simulink model "VSC_GFo_Variable_Frequency_LCL"  (R2017b)
settings: Solver=ode1  StartTime=0.0  StopTime=8  FixedStep=Time_Step  MaxStep=1e-5  RelTol=1e-3
PreLoadFcn:
  | VSC_GFo_Init;
InitFcn:
  | VSC_GFo_Init;
values from neighbouring files (symbols this model uses):
  DX_DR = 5    [VSC_GFo_Init.m]
  fb = fn    (= 50)    [VSC_GFo_Init.m]    (also in VSC_GFo_Init_v1.m; VSC_GFo_Init_wi_LCL.m)
  fn = 50    [VSC_GFo_Init.m]    (also in VSC_GFo_Init_v1.m; VSC_GFo_Init_wi_LCL.m)
  GRD00_H = 5    [VSC_GFo_Init.m]    (also in VSC_GFo_Init_v1.m; VSC_GFo_Init_wi_LCL.m)
  GRD00_Lg = GRD00_Xg/wb    (= 0.0254647908947)    [VSC_GFo_Init.m]    (also in VSC_GFo_Init_v1.m; VSC_GFo_Init_wi_LCL.m)
  GRD00_R = 4/100    (= 0.04)    [VSC_GFo_Init.m]    (also in VSC_GFo_Init_v1.m; VSC_GFo_Init_wi_LCL.m)
  GRD00_Rg = GRD00_Rg_pu*GRD00_Zb    (= 0.8)    [VSC_GFo_Init.m]    (also in VSC_GFo_Init_v1.m; VSC_GFo_Init_wi_LCL.m)
  GRD00_TD = 6    [VSC_GFo_Init.m]    (also in VSC_GFo_Init_v1.m = 2; VSC_GFo_Init_wi_LCL.m = 2)
  GRD00_TN = 1    [VSC_GFo_Init.m]    (also in VSC_GFo_Init_v1.m; VSC_GFo_Init_wi_LCL.m)
  GRD00_Ub = GRD00_Un    (= 400000)    [VSC_GFo_Init.m]    (also in VSC_GFo_Init_v1.m; VSC_GFo_Init_wi_LCL.m)
  I_thresh_pu = 1    [VSC_GFo_Init.m]
  Kp_Rvi_pu = 0.676    [VSC_GFo_Init.m]
  Time_Step = 40e-6    (= 4e-05)    [VSC_GFo_Init.m]    (also in VSC_GFo_Init_v1.m; VSC_GFo_Init_wi_LCL.m)
  VSC01_Cf = VSC01_Cf_pu * VSC01_Cb    [VSC_GFo_Init.m]    (also in VSC_GFo_Init_wi_LCL.m)
  VSC01_Cf_pu = 0.066    [VSC_GFo_Init.m]    (also in VSC_GFo_Init_wi_LCL.m)
  VSC01_Delta_P_Time_Step = 0.2    [VSC_GFo_Init.m]    (also in VSC_GFo_Init_v1.m; VSC_GFo_Init_wi_LCL.m)
  VSC01_Delta_P_Value = 0    [VSC_GFo_Init.m]    (also in VSC_GFo_Init_v1.m = 0.2; VSC_GFo_Init_wi_LCL.m = 0.2)
  VSC01_Lf = VSC01_Lf_pu * VSC01_Lb    [VSC_GFo_Init.m]    (also in VSC_GFo_Init_wi_LCL.m)
  VSC01_Lf_pu = 0.15    [VSC_GFo_Init.m]    (also in VSC_GFo_Init_wi_LCL.m)
  VSC01_Lt_pu = 0.15    [VSC_GFo_Init.m]    (also in VSC_GFo_Init_v1.m; VSC_GFo_Init_wi_LCL.m)
  VSC01_mp1 = 0.0043    [VSC_GFo_Init.m]    (also in VSC_GFo_Init_v1.m; VSC_GFo_Init_wi_LCL.m)
  VSC01_mp2 = 0.003    [VSC_GFo_Init.m]    (also in VSC_GFo_Init_v1.m = 0.0033; VSC_GFo_Init_wi_LCL.m = 0.0033)
  VSC01_mp3 = 0.04    [VSC_GFo_Init.m]    (also in VSC_GFo_Init_v1.m; VSC_GFo_Init_wi_LCL.m)
  VSC01_Pn = 1000 * 1e6    (= 1000000000)    [VSC_GFo_Init.m]    (also in VSC_GFo_Init_v1.m; VSC_GFo_Init_wi_LCL.m)
  VSC01_R = 4/100    (= 0.04)    [VSC_GFo_Init.m]    (also in VSC_GFo_Init_v1.m; VSC_GFo_Init_wi_LCL.m)
  VSC01_Rf = VSC01_Rf_pu * VSC01_Zb    [VSC_GFo_Init.m]    (also in VSC_GFo_Init_wi_LCL.m)
  VSC01_Rf_pu = 0.005    [VSC_GFo_Init.m]    (also in VSC_GFo_Init_wi_LCL.m)
  VSC01_Rt_pu = 0.005    [VSC_GFo_Init.m]    (also in VSC_GFo_Init_v1.m; VSC_GFo_Init_wi_LCL.m)
  VSC01_Rv = 0.09    [VSC_GFo_Init.m]    (also in VSC_GFo_Init_v1.m; VSC_GFo_Init_wi_LCL.m)
  VSC01_Sn = VSC01_Pn/VSC01_cosPhi_n    [VSC_GFo_Init.m]    (also in VSC_GFo_Init_v1.m; VSC_GFo_Init_wi_LCL.m)
  VSC01_T1 = 0.121    [VSC_GFo_Init.m]    (also in VSC_GFo_Init_v1.m; VSC_GFo_Init_wi_LCL.m)
  VSC01_T2 = 0.022    [VSC_GFo_Init.m]    (also in VSC_GFo_Init_v1.m; VSC_GFo_Init_wi_LCL.m)
  VSC01_Tr_PLL = 0.010    (= 0.01)    [VSC_GFo_Init.m]    (also in VSC_GFo_Init_v1.m; VSC_GFo_Init_wi_LCL.m)
  VSC01_Udc_n = 640 * 1e3    (= 640000)    [VSC_GFo_Init.m]    (also in VSC_GFo_Init_v1.m; VSC_GFo_Init_wi_LCL.m)
  VSC01_Udcb = VSC01_Udc_n    (= 640000)    [VSC_GFo_Init.m]    (also in VSC_GFo_Init_v1.m; VSC_GFo_Init_wi_LCL.m)
  VSC01_Un1 = 320 * 1e3    (= 320000)    [VSC_GFo_Init.m]    (also in VSC_GFo_Init_v1.m; VSC_GFo_Init_wi_LCL.m)
  VSC01_Un2 = 400 * 1e3    (= 400000)    [VSC_GFo_Init.m]    (also in VSC_GFo_Init_v1.m; VSC_GFo_Init_wi_LCL.m)
  VSC01_W_LF = 60    [VSC_GFo_Init.m]    (also in VSC_GFo_Init_v1.m; VSC_GFo_Init_wi_LCL.m)
  VSC01_wc1 = wb/10    (= 31.4159265359)    [VSC_GFo_Init.m]    (also in VSC_GFo_Init_v1.m; VSC_GFo_Init_wi_LCL.m)
  VSC01_wc2 = 33.3    [VSC_GFo_Init.m]    (also in VSC_GFo_Init_v1.m; VSC_GFo_Init_wi_LCL.m)
  VSC01_wc3 = 2.5    [VSC_GFo_Init.m]    (also in VSC_GFo_Init_v1.m; VSC_GFo_Init_wi_LCL.m)
undefined symbols (not defined in the file or in its folder): C_line, VSC01_id0
libraries: powerlib x29, simulink x1, powerlib_meascontrol x1
(part 1 of 2)
settings Model: Creator=Frederic_Colas  LastModifiedBy=Frederic_Colas
settings OptimizationCC: LifeSpan=inf
settings DebuggingCC: UnconnectedInputMsg=none  UnconnectedOutputMsg=none  UnconnectedLineMsg=none  SFExecutionAtInitializationDiag=none
settings HardwareCC: ProdBitPerSizeT=32  ProdBitPerPtrDiffT=32  ProdWordSize=32  ProdHWDeviceType=Specified
settings CodeAppCC: StateflowObjectComments=on
settings SimscapeCC: SimscapeNormalizeSystem=off

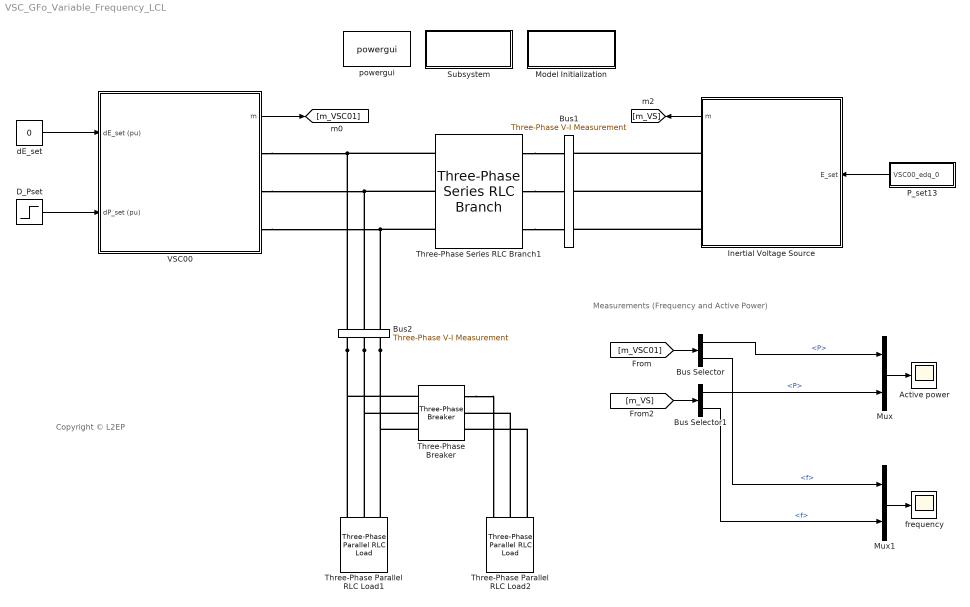
== system VSC_GFo_Variable_Frequency_LCL ==
  note: Measurements (Frequency and Active Power)
  note: Copyright © L2EP
  Active power : Scope
  Bus Selector : BusSelector  OutputSignals=control.P,control.f
  Bus Selector1 : BusSelector  OutputSignals=P,f
  Bus1 : powerlib/Measurements/Three-Phase V-I Measurement  VoltageMeasurement=no  SetLabelV=off  LabelV=Vabc  Vpu=off  VpuLL=off  CurrentMeasurement=no  SetLabelI=off  LabelI=Iabc  Ipu=off  Pbase=1e9  Vbase=VSC01_Un2  OutputType=Complex  PhasorSimulation=off  PSBequivalent=0
  "Bus2 " : powerlib/Measurements/Three-Phase V-I Measurement  VoltageMeasurement=no  SetLabelV=off  LabelV=Vabc  Vpu=off  VpuLL=off  CurrentMeasurement=no  SetLabelI=off  LabelI=Iabc  Ipu=off  Pbase=100e6  Vbase=500e3  OutputType=Complex  PhasorSimulation=off  PSBequivalent=0
  D_Pset : Step  Time=VSC01_Delta_P_Time_Step  After=VSC01_Delta_P_Value  SampleTime=0
  Inertial Voltage Source : Subsystem  mask(Inertial_Voltage_source){fb=fb, Sc=1e9, Ub=GRD00_Ub, H_eq=GRD00_H, Droop=GRD00_R, TN=GRD00_TN, TD=GRD00_TD, P0=-0.39869}
      mask prompts: fb "Nominal Frequency (Hz)"; Sc "Nominal Power (VA)"; Ub "Nominal Voltage (V)"; H_eq "Inertial Constant H (s)"; Droop "Droop Gain"; TN "Lead Time Constant"; TD "Lag Time Constant"; P0 "Initial Power"
      mask init:
      | % Update Name of LF bus for internal purpose
      |     NameStr = [get_param(gcb,'Name')];% '_LF'];
      |     set_param([gcb '/Load Flow Bus'],'ID',NameStr);
      | 
      | % Base values
      |     wb=2*pi*fb;
      |     Ib=Sc/(sqrt(3)*Ub);
      |     Vb=Ub/sqrt(3);
      |     e0=Vb;
      |     Theta_e0=0;
      |     P0_VS = P0;
      |   
      | % Parameters
      |     R=Droop;
      mask DialogControl Container5 Prompt: Nominal Values
      mask DialogControl Container16 Prompt: Network Time Constants
  Model Initialization : Subsystem  mask(Model Functions){InitFcnX=VSC_GFo_Init;, prel=on, posl=off, inif=on, strf=off}
      mask prompts: InitFcnX "Initialisation"; prel "Preload Function"; posl "PostLoad Function"; inif "InitFcn"; strf "StartFcn"
      mask init:
      | currentBlock = gcb;
      | root = bdroot(currentBlock);
      | 
      | if ~strcmp(get_param(root,'BlockDiagramType'),'library')
      |     if prel==1
      |         set_param(root, 'PreLoadFcn', InitFcnX);
      |     else
      |         set_param(root, 'PreLoadFcn', '');
      |     end
      |     if inif==1
      |         set_param(root, 'InitFcn', InitFcnX);
      |     else
      |         set_param(root, 'InitFcn', '');
      |     end
      |     if strf==1
      |         set_param(root, 'StartFcn', InitFcnX);
      |     else
      |         set_param(root, 'StartFcn', '');
      |     end
      |     if posl==1
      |         set_param(root, 'PostLoadFcn', InitFcnX);
      |     else
      |         set_param(root, 'PostLoadFcn', '');
      |     end
      | end
      | 
      | pos = get_param(currentBlock, 'Position');
      | width = pos(3) - pos(1); height = pos(4) - pos(2);
      | txt = [ upper(root) '\n' '- InitFcn. . . . . '  get_param(root, 'InitFcn') ];
      settings: CopyFcn=set_param(gcb,'LinkStatus','none')
      mask Display:
      | %text(5, height*0.5, txt, 'horizontalAlignment', 'left', 'verticalAlignment', 'middle') ;
      | color('blue'),disp('Initialization Function\nParameters')
  Mux : Mux  Inputs=2
  Mux1 : Mux  Inputs=2
  P_set13 : Subsystem
  Subsystem : Subsystem
      settings: OpenFcn=LoadFlow_VSC
      mask Display: color('blue'),disp('Update Loadflow')
  Three-Phase Parallel RLC Load1 : powerlib/Elements/Three-Phase Parallel RLC Load  LConnTagsString=A|B|C  Configuration=Y (grounded)  NominalVoltage=GRD00_Un  Vabc=[1e3 1e3 1e3]  Vabcp=[1e3 1e3 1e3]  NominalFrequency=fb  UnbalancedPower=off  ActivePower=100e6  InductivePower=0  CapacitivePower=0  Pabc=[10e3 9e3 11e3]  QLabc=[100 90 110]  QCabc=[100 90 110]  Pabcp=[10e3 9e3 11e3]  QLabcp=[100 90 110]  QCabcp=[100 90 110]  Measurements=None  LoadType=constant Z
  Three-Phase Parallel RLC Load2 : powerlib/Elements/Three-Phase Parallel RLC Load  LConnTagsString=A|B|C  Configuration=Y (grounded)  NominalVoltage=GRD00_Un  Vabc=[1e3 1e3 1e3]  Vabcp=[1e3 1e3 1e3]  NominalFrequency=fb  UnbalancedPower=off  ActivePower=400e6  InductivePower=0  CapacitivePower=0  Pabc=[10e3 9e3 11e3]  QLabc=[100 90 110]  QCabc=[100 90 110]  Pabcp=[10e3 9e3 11e3]  QLabcp=[100 90 110]  QCabcp=[100 90 110]  Measurements=None  LoadType=constant Z
  Three-Phase Series RLC Branch1 : powerlib/Elements/Three-Phase Series RLC Branch  LConnTagsString=A|B|C  RConnTagsString=A|B|C  BranchType=RL  Resistance=GRD00_Rg  Inductance=GRD00_Lg  Capacitance=1e-6  Measurements=None
  Three-Phase Breaker : powerlib/Elements/Three-Phase Breaker  InitialState=open  SwitchA=on  SwitchB=on  SwitchC=on  SwitchTimes=[1 60]  External=off  BreakerResistance=0.01  SnubberResistance=1e6  SnubberCapacitance=inf  Measurements=None
  VSC00 : Subsystem  mask(VSC){fb=fb, Sn=VSC01_Sn, Pn=VSC01_Pn, Un1=VSC01_Un1, Un2=VSC01_Un2, Rt_pu=VSC01_Rt_pu, Lt_pu=VSC01_Lt_pu, Rm_pu=500, Lm_pu=0, Lf_pu=VSC01_Lf_pu, Rf_pu=VSC01_Rf_pu, Cf_pu=VSC01_Cf_pu, Tr_PLL=VSC01_Tr_PLL, Val_Freq_Support=on, Val_gamma=on, R_percent=VSC01_R, Rv=VSC01_Rv, W_TVR=VSC01_W_LF, gainpopup=3, wc1=VSC01_wc1, mp1=VSC01_mp1, wc2=VSC01_wc2, mp2=VSC01_mp2, wc3=VSC01_wc3, mp3=VSC01_mp3, T1=VSC01_T1, T2=VSC01_T2, LFpopup=PQ, P0=0.5, Q0=2.0738e-05, V0=1, Theta0=1.1424, innercontrol=1, Ki_i=1.19, Kp_i=0.73, Kp_v=0.52, Ki_v=1.16, Kffv=1, Kffi=1, I_max=1.25}
      mask prompts: fb "Nominal Frequency (Hz)"; Sn "Nominal Apparent Power (VA)"; Pn "Nominal Power (W)"; Un1 "VSC side Nominal Ph-Ph Voltage (V)"; Un2 "Grid side Nominal Ph-Ph Voltage (V)"; Rt_pu "R (pu)"; Lt_pu "L (pu)"; Rm_pu "Rm (pu)"; Lm_pu "Lm (pu)"; Lf_pu "Lf (pu)"; Rf_pu "Rf (pu)"; Cf_pu "Cf (pu)"; Tr_PLL "Time response (s)"; Val_Freq_Support "Frequency Support"; Val_gamma "gamma activation"; R_percent "Droop Gain (%)"; Rv "Damping Resistance (Rv)"; W_TVR "Dr filter"; gainpopup "Strategy"; wc1 "wc"; mp1 "mp"; wc2 "wc"; mp2 "mp"; wc3 "wc"; mp3 "mp"; P0 "Initial Active Power (pu)"; Q0 "Initial Reactive Power (pu)"; V0 "Initial Voltage (pu)"; Theta0 "Initial Angle (°)"; innercontrol "Strategy"
      mask init:
      | % Update Name of LF bus for internal purpose
      |     NameStr = [get_param(gcb,'Name')];% '_LF'];
      |     set_param([gcb '/Load Flow Bus'],'ID',NameStr);
      |     %disp(NameStr);
      |     
      | % Increase size of Mask dialog box
      |    % pause(0.1);
      |     
      |     
      | % Base values
      |     %Un = Un1;
      |     Pb = Pn;
      |     cos_phi_n = Pn/Sn;
      |     Sb = Pb/cos_phi_n;
      |     %Ub = Un;
      |     Vn = Un1/sqrt(3);
      |     Vb = Vn;
      |     %Ib = Sb / Ub;
      |     Ib = Sb / (3*Vb);
      |     Zb = (3*Vb^2)/Sb;
      |     wb = 2*pi*fb;
      |     Lb = Zb/wb;
      |     Cb = 1/(Zb*wb);
      |   
      | % PLL derivation of the parameters
      |     wn_PLL=5/Tr_PLL;
      |     zeta_PLL = 1;
      |     Kp_PLL_pu = 2*zeta_PLL*wn_PLL/wb;
      |     Ki_PLL_pu = wn_PLL^2/wb;
      |     
      | % Set the chosen strategy
      |     Chosen_Strategy = str2double(gainpopup);
      |     
      | % Set the frequency droop gain
      |     R = R_percent;
      | 
      | % Compute Initial Voltage of VSC 
      | %   from steady-state output transformer model and Loadflow result
      |     if (LFpopup == 'PQ')
      |         V0 = 1;
      |     end
      |         
      |     R1_pu = Rt_pu/2;
      |     L1_pu = Lt_pu/2;
      |     R2_pu = Rt_pu/2;
      |     L2_pu = Lt_pu/2;
      |     X1_pu = L1_pu;
      |     X2_pu = L2_pu;
      |     Xm_pu = Lm_pu;
      |     
      |     Zm_pu = 1/(1/Rm_pu);
      | 
      |     S0=P0+1i*Q0;
      |     I2 = conj(S0)/(V0);
      | 
      |     Vm = (R2_pu+1i*X2_pu)*I2 + V0;
      |     Im = Vm/Zm_pu;
      | 
      |     I1 = I2 + Im;
      |     V1 = (R1_pu+1i*X1_pu) * I1 + Vm;
      | 
      |     Vvsc0 = abs(V1);
      |    % disp(Vvsc0*1000)
      |     Theta_vsc0 = angle(V1) * 180/pi+Theta0;
      |         
      |     %vd0=Vvsc0*cos(Theta0*2*pi/180);
      |     %vq0=Vvsc0*sin(Theta0*2*pi/180); 
      |  
      |     %Va0 = Vvsc0*sqrt(2)*Ub/sqrt(3)*sin(Theta_vsc0*pi/180);
      |     %Vb0 = Vvsc0*sqrt(2)*Ub/sqrt(3)*sin(Theta_vsc0*pi/180-2*pi/3);
      |     %Vc0 = Vvsc0*sqrt(2)*Ub/sqrt(3)*sin(Theta_vsc0*pi/180+2*pi/3);
      |     
      |     Va0 = Vvsc0*sqrt(2)*Vb*sin(Theta_vsc0*pi/180);
      |     Vb0 = Vvsc0*sqrt(2)*Vb*sin(Theta_vsc0*pi/180-2*pi/3);
      |     Vc0 = Vvsc0*sqrt(2)*Vb*sin(Theta_vsc0*pi/180+2*pi/3);
      |     
      | % Generate string to display LF results on Mask
      |     %str_tmp = fprintf("Vvsc0 = %d, Theta_vsc0 = %d°",Vvsc0,Theta_vsc0);
      |     mo = get_param(gcb,'MaskObject');
      |     mo.getDialogControl('LF_vsc_str').Prompt = ['V0 = ', num2str(Vvsc0),' pu, Angle = ', num2str(Theta_vsc0),'°'];
      |     mo.getDialogControl('LF_pcc_str').Prompt = ['V0 = ', num2str(V0),' pu, Angle = ', num2str(Theta0),'°'];
      |     mo.getDialogControl('LF_pcc_Power_str').Prompt = ['P0 = ', num2str(P0),' pu, Q0 = ', num2str(Q0),' pu'];
      |     %set_param([gcb],'LF_str',str_tmp);
      |  %GRD00_Theta0 = Theta0;
      |  %P0 = 200e6;
      |  %Q0 = 0;
      |  % Initial current values of VSC (dq pu) 
      |  %id0 =(P0*vd0+Q0*vq0)/(vd0^2+vq0^2) * 1/Ib; %
      |  %iq0 =(P0*vq0-Q0*vd0)/(vd0^2+vq0^2) * 1/Ib; %Initial current in the connexion inductance
      settings: OpenFcn=|
      | NameStr = get_param(gcb,'Name');
      | open_system(gcbh, 'Mask');
      | 
      | h2AllOpenDlgs = DAStudio.ToolRoot.getOpenDialogs;
      | 
      | for i=1:length(h2AllOpenDlgs)
      |     try
      |          %disp(h2AllOpenDlgs(i).getSource.getBlock.Name);
      |         Dialog_block_name = h2AllOpenDlgs(i).getSource.getBlock.Name;
      |          %strcmp(Dialog_block_name, NameStr),
      |         if (strcmp(h2AllOpenDlgs(i).getSource.getBlock.Name, NameStr))
      |             iPos = h2AllOpenDlgs(i).position;
      |             h2AllOpenDlgs(i).position = [iPos(1)   iPos(2)   iPos(3)*1.6   iPos(4)];
      |         end
      |     end
      | end
      mask TypeOptions gainpopup: 1 | 2 | 3
      mask Callback gainpopup:
      | % Get the mask parameter values. This is a cell
      | %   array of character vectors.
      | maskStr = get_param(gcb,'gainpopup');
      | p=Simulink.Mask.get(gcb);
      | 
      | % The pop-up menu is the first mask parameter.
      | %   Check the value selected in the pop-up
      | if strcmp(maskStr,'1'),
      | 
      |     % Set the visibility of both parameters on when
      |     %   User-defined is selected in the pop-up.
      |     p.getDialogControl('Param_Strat_1').Visible='on';
      |     p.getDialogControl('Param_Strat_2').Visible='off';
      |     p.getDialogControl('Param_Strat_3').Visible='off';
      | 
      | 
      | elseif strcmp(maskStr,'2'),
      | 
      |     % Set the visibility of both parameters on when
      |     %   User-defined is selected in the pop-up.
      |     p.getDialogControl('Param_Strat_1').Visible='off';
      |     p.getDialogControl('Param_Strat_2').Visible='on';
      |     p.getDialogControl('Param_Strat_3').Visible='off';
      | 
      | 
      |     % Turn off the visibility of the Value field
      |     %   when User-defined is not selected.
      | elseif strcmp(maskStr,'3'),
      | 
      |     % Set the visibility of both parameters on when
      |     %   User-defined is selected in the pop-up.
      |     p.getDialogControl('Param_Strat_1').Visible='off';
      |     p.getDialogControl('Param_Strat_2').Visible='off';
      |     p.getDialogControl('Param_Strat_3').Visible='on';
      | 
      | else
      | 
      |     % Set the visibility of both parameters on when
      |     %   User-defined is selected in the pop-up.
      |     p.getDialogControl('Param_Strat_1').Visible='off';
      |     p.getDialogControl('Param_Strat_2').Visible='off';
      |     p.getDialogControl('Param_Strat_3').Visible='off';
      | 
      | end
      mask TypeOptions LFpopup: Swing | PQ | PV
      mask Callback LFpopup:
      | % Get the mask parameter values. This is a cell
      | %   array of character vectors.
      | maskStr = get_param(gcb,'LFpopup');
      | p=Simulink.Mask.get(gcb);
      | 
      | % The pop-up menu is the first mask parameter.
      | %   Check the value selected in the pop-up
      | if strcmp(maskStr,'Swing'),
      | 
      |     % Set the visibility of both parameters on when
      |     %   User-defined is selected in the pop-up.
      |     p.getParameter('P0').Visible='off';
      |     p.getParameter('Q0').Visible='off';
      |     p.getParameter('V0').Visible='on';
      |     p.getParameter('Theta0').Visible='on';
      |     set_param([gcb '/Source_For_LF'],'BusType','swing');
      | 
      | elseif strcmp(maskStr,'PQ'),
      | 
      |     % Set the visibility of both parameters on when
      |     %   User-defined is selected in the pop-up.
      |     p.getParameter('P0').Visible='on';
      |     p.getParameter('Q0').Visible='on';
      |     p.getParameter('V0').Value='1';
      |     set_param(gcb,'V0','1');
      |     p.getParameter('V0').Visible='off';
      |     p.getParameter('Theta0').Visible='off';
      |     set_param([gcb '/Source_For_LF'],'BusType','PQ');
      | 
      |     % Turn off the visibility of the Value field
      |     %   when User-defined is not selected.
      | else
      | 
      |     % Set the visibility of both parameters on when
      |     %   User-defined is selected in the pop-up.
      |     p.getParameter('P0').Visible='on';
      |     p.getParameter('Q0').Visible='off';
      |     p.getParameter('V0').Visible='on';
      |     p.getParameter('Theta0').Visible='off';
      |     set_param([gcb '/Source_For_LF'],'BusType','PV');
      | 
      | end
      mask TypeOptions innercontrol: 1
      mask Callback innercontrol:
      | % Get the mask parameter values. This is a cell
      | %   array of character vectors.
      | maskStr = get_param(gcb,'innercontrol');
      | p=Simulink.Mask.get(gcb);
      | 
      | % The pop-up menu is the first mask parameter.
      | %   Check the value selected in the pop-up
      | if strcmp(maskStr,'1'),
      | 
      |     % Set the visibility of both parameters on when
      |     %   User-defined is selected in the pop-up.
      |     p.getDialogControl('Param_Strat_11').Visible='on';
      | 
      | 
      | else
      | 
      |     % Set the visibility of both parameters on when
      |     %   User-defined is selected in the pop-up.
      |     p.getDialogControl('Param_Strat_11').Visible='on';
      | 
      | end
      mask DialogControl Nominal_Param Prompt: Nominal Value
      mask DialogControl Container20 Prompt: Output Transformer and filter
      mask DialogControl Container31 Prompt: Transformer
      mask DialogControl Container32 Prompt: Filter
      mask DialogControl Control_Param Prompt: Control Parameter
      mask DialogControl Container13 Prompt: PLL
      mask DialogControl Container14 Prompt: Frequency Support
      mask DialogControl Container15 Prompt: Transient Virtual Resistor
      mask DialogControl Container18 Prompt: Control Strategy
      mask DialogControl Title_Strat_1 Prompt: Strategy 1
      mask DialogControl Title_Strat_2 Prompt: Strategy 2
      mask DialogControl Title_Strat_3 Prompt: Strategy 3
      mask DialogControl LF_Param Prompt: Loadflow
      mask DialogControl Control4 Prompt: Initial Operating Point
      mask DialogControl Container24 Prompt: VSC side
      mask DialogControl LF_vsc_str Prompt: V0 = 1.0053 pu, Angle = 5.4294°
      mask DialogControl Container25 Prompt: PCC
      mask DialogControl LF_pcc_str Prompt: V0 = 1 pu, Angle = 1.1424°
      mask DialogControl LF_pcc_Power_str Prompt: P0 = 0.5 pu, Q0 = 2.0738e-05 pu
      mask DialogControl UpdateLoadflow Prompt: Update Loadflow
      mask DialogControl UpdateLoadflow Callback: Load_Flow_VSC
      mask DialogControl Container21 Prompt: Inner control
      mask DialogControl Title_Strat_11 Prompt: Cascaded_control
  dE_set : Constant  Value=0
  frequency : Scope
  powergui : powerlib/powergui  Priority=1  SimulationMode=Discrete  SampleTime=Time_Step  frequency=60  Iterations=50  frequencyindice=50  Pbase=1000e6  ErrMax=1e-4  UnitsV=kV  UnitsW=MW  buscounter=0  FunctionMessages=off  echomessages=off  EnableUseOfTLC=off  CurrentSourceSwitches=off  DisableSnubberDevices=off  DisableRonSwitches=off  DisableVfSwitches=off  DisplayEquations=off  SolverType=Tustin/Backward Euler (TBE)  Interpol=off  ExternalGateDelay=off  methode=off  Ts=100  x0status=blocks  SPID=on  SwTol=0  HookPort=off  RestoreLinks=warning  ResistiveCurrentMeasurement=off  Frange=[0:2:500]  Ylog=off  Xlog=on  ShowGrid=off  save=off  variable=ZData  structure=0  ZoomFFT=off  StartTime=0.0  cycles=1  DisplayStyle=1  fundamental=60  FreqAxis=off  MaxFrequency=1000  frequencyindicesteady=1  RmsSteady=1  display=off
  wires:
  VSC00/1(m) -> [m_VSC01]
  Inertial Voltage Source/1("m ") -> [m_VS]
  P_set13/1(VSC00_edq_0) -> Inertial Voltage Source/1(E_set)
  Mux1/1 -> frequency/1
  [m_VS] -> Bus Selector1/1
  [m_VSC01] -> Bus Selector/1
  Bus Selector1/2 -> Mux1/2  "<f>"
  Mux/1 -> Active power/1
  Bus Selector1/1 -> Mux/2  "<P>"
  Bus Selector/2 -> Mux1/1  "<f>"
  Bus Selector/1 -> Mux/1  "<P>"
  D_Pset/1 -> VSC00/2(dP_set (pu))
  dE_set/1 -> VSC00/1(dE_set (pu))
  connections:
  Three-Phase Series RLC Branch1/LConn1 -- VSC00/RConn1 -- "Bus2 "/LConn3
  Three-Phase Series RLC Branch1/RConn2 -- Bus1/LConn2
  Three-Phase Series RLC Branch1/LConn3 -- VSC00/RConn3 -- "Bus2 "/LConn1
  Three-Phase Series RLC Branch1/LConn2 -- VSC00/RConn2 -- "Bus2 "/LConn2
  Three-Phase Series RLC Branch1/RConn3 -- Bus1/LConn3
  Three-Phase Series RLC Branch1/RConn1 -- Bus1/LConn1
  Inertial Voltage Source/RConn1 -- Bus1/RConn1
  Inertial Voltage Source/RConn2 -- Bus1/RConn2
  Inertial Voltage Source/RConn3 -- Bus1/RConn3
  "Bus2 "/RConn1 -- Three-Phase Breaker/LConn3 -- Three-Phase Parallel RLC Load1/LConn3
  "Bus2 "/RConn3 -- Three-Phase Breaker/LConn1 -- Three-Phase Parallel RLC Load1/LConn1
  "Bus2 "/RConn2 -- Three-Phase Breaker/LConn2 -- Three-Phase Parallel RLC Load1/LConn2
  Three-Phase Breaker/RConn1 -- Three-Phase Parallel RLC Load2/LConn1
  Three-Phase Parallel RLC Load2/LConn3 -- Three-Phase Breaker/RConn3
  Three-Phase Parallel RLC Load2/LConn2 -- Three-Phase Breaker/RConn2

== system VSC_GFo_Variable_Frequency_LCL/Inertial Voltage Source ==
  E_set : Inport
  Bus00 : powerlib/Measurements/Three-Phase V-I Measurement  VoltageMeasurement=phase-to-ground  SetLabelV=off  LabelV=Vabc  Vpu=off  VpuLL=off  CurrentMeasurement=yes  SetLabelI=off  LabelI=Iabc  Ipu=off  Pbase=100e6  Vbase=500e3  OutputType=Complex  PhasorSimulation=off  PSBequivalent=0
  Load Flow Bus : powerlib/Measurements/Load Flow Bus  LConnTagsString=a  Phases=single  Connectors=on one side  ID=Inertial Voltage Source  Vbase=Ub  Vref=1  Vangle=0  VLF=1  VLFb=1  VLFc=1  angleLF=0  angleLFb=0  angleLFc=0
      settings: SourceProductName=Simscape Power Systems
  Mean_model : Subsystem
  Simplified SG : Subsystem
  Source_For_LF : powerlib/Electrical Sources/Three-Phase Source  Commented=on  InternalConnection=Yg  VoltagePhases=off  Voltage=(400000)*1  PhaseAngle=0  Voltage_phases=[25e3 25e3 25e3]/sqrt(3)  PhaseAngles_phases=[0 -120 +120]  Frequency=fb  NonIdealSource=on  SpecifyImpedance=off  Resistance=0  Inductance=0  ShortCircuitLevel=100e6  BaseVoltage=GRD00_Un  XRratio=7  BusType=swing  Pref=P0  Qref=Q0  Prefabc=[10e3, 10e3, 10e3]  Qrefabc=[0, 0, 0]  Qmin=-inf  Qmax=inf
  A : PMIOPort  Port=1  Side=Right
  B : PMIOPort  Port=2  Side=Right
  C : PMIOPort  Port=3  Side=Right
  "m " : Outport
  wires:
  [GRD00_U_abc] -> Simplified SG/1(eg_mes)
  E_set/1 -> Simplified SG/3(E_set)
  Simplified SG/1(vg_abc) -> Mean_model/1(u_abc)
  [GRD00_i_abc] -> Simplified SG/2(ig_mes)
  Simplified SG/2(m) -> "m "/1
  Bus00/1 -> [GRD00_U_abc]
  Bus00/2 -> [GRD00_i_abc]
  connections:
  Source_For_LF/RConn3 -- Bus00/LConn3 -- Mean_model/RConn3
  Source_For_LF/RConn2 -- Bus00/LConn2 -- Mean_model/RConn2
  Source_For_LF/RConn1 -- Load Flow Bus/LConn1 -- Bus00/LConn1 -- Mean_model/RConn1
  A/RConn1 -- Bus00/RConn1
  B/RConn1 -- Bus00/RConn2
  C/RConn1 -- Bus00/RConn3

== system VSC_GFo_Variable_Frequency_LCL/Model Initialization ==

== system VSC_GFo_Variable_Frequency_LCL/P_set13 ==
  Mux : Mux  Inputs=2
  ed1 : Constant  Value=0
  eq1 : Constant
  VSC00_edq_0 : Outport
  wires:
  Mux/1 -> VSC00_edq_0/1
  eq1/1 -> Mux/1
  ed1/1 -> Mux/2

== system VSC_GFo_Variable_Frequency_LCL/Subsystem ==

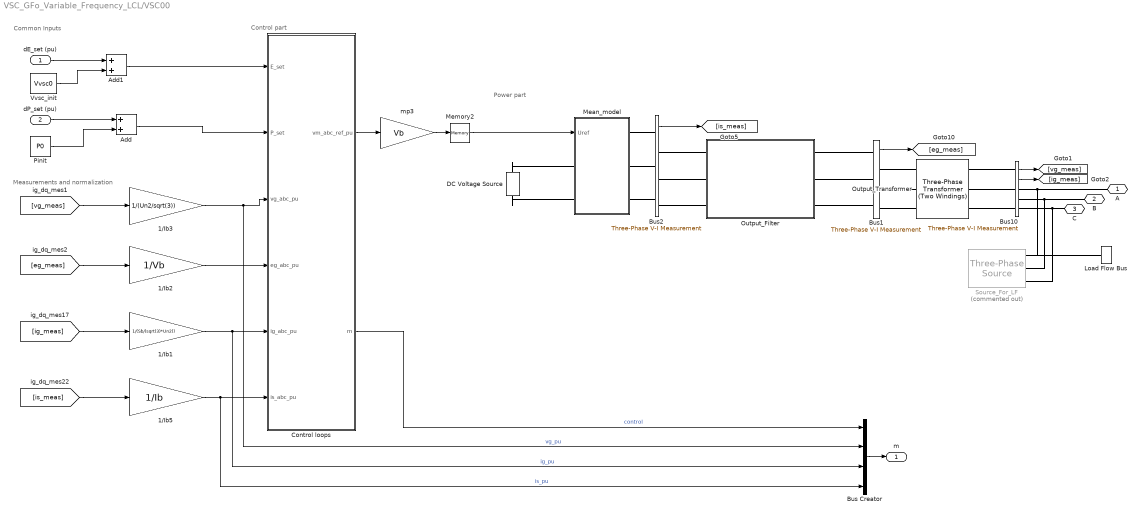
== system VSC_GFo_Variable_Frequency_LCL/VSC00 ==
  note: Control part
  note: Measurements and normalization
  note: Power part
  note: Common Inputs
  dE_set (pu) : Inport
  dP_set (pu) : Inport  Port=2
  1/Ib1 : Gain  Gain=1/(Sb/(sqrt(3)*Un2))
  1/Ib2 : Gain  Gain=1/Vb
  1/Ib3 : Gain  Gain=1/(Un2/sqrt(3))
  1/Ib5 : Gain  Gain=1/Ib
  Add : Sum
  Add1 : Sum
  Bus Creator : BusCreator  Inputs=4
  Bus1 : powerlib/Measurements/Three-Phase V-I Measurement  VoltageMeasurement=phase-to-ground  SetLabelV=off  LabelV=Vabc  Vpu=off  VpuLL=off  CurrentMeasurement=no  SetLabelI=off  LabelI=Iabc  Ipu=off  Pbase=100e6  Vbase=500e3  OutputType=Complex  PhasorSimulation=off  PSBequivalent=0
  Bus10 : powerlib/Measurements/Three-Phase V-I Measurement  VoltageMeasurement=phase-to-ground  SetLabelV=off  LabelV=Vabc  Vpu=off  VpuLL=off  CurrentMeasurement=yes  SetLabelI=off  LabelI=Iabc  Ipu=off  Pbase=100e6  Vbase=500e3  OutputType=Complex  PhasorSimulation=off  PSBequivalent=0
  Bus2 : powerlib/Measurements/Three-Phase V-I Measurement  VoltageMeasurement=no  SetLabelV=off  LabelV=Vabc  Vpu=off  VpuLL=off  CurrentMeasurement=yes  SetLabelI=off  LabelI=Iabc  Ipu=off  Pbase=100e6  Vbase=500e3  OutputType=Complex  PhasorSimulation=off  PSBequivalent=0
  Control loops : Subsystem
  DC Voltage Source : powerlib/Electrical Sources/DC Voltage Source  Amplitude=VSC01_Udc_n  Measurements=Voltage
  Load Flow Bus : powerlib/Measurements/Load Flow Bus  LConnTagsString=a  Phases=single  Connectors=on one side  ID=VSC00  Vbase=Un2  Vref=V0  Vangle=Theta0  VLF=1.002  VLFb=1  VLFc=1  angleLF=1.142  angleLFb=0  angleLFc=0
      settings: SourceProductName=Simscape Power Systems
  Mean_model : Subsystem
  Memory2 : Memory  InitialCondition=[Va0 Vb0 Vc0]
  Output_Filter : Subsystem  mask{Lf=VSC01_Lf, Rf=VSC01_Rf, Cf=VSC01_Cf}
      mask prompts: Lf "Filter inductance [H]"; Rf "Filter resistance [R]"; Cf "Filter capacitance [F]"
  Output_Transformer : powerlib/Elements/Three-Phase Transformer (Two Windings)  Winding1Connection=Yg  Winding2Connection=Yg  CoreType=Three single-phase transformers  SetSaturation=off  Hysteresis=off  DataFile='hysteresis'  SetInitialFlux=off  Measurements=None  UNITS=pu  NominalPower=[Sn , fn ]  Winding1=[Un1 , Rt_pu/2 , Lt_pu/2]  Winding2=[Un2 , Rt_pu/2 , Lt_pu/2]  Rm=Rm_pu  Lm=Lm_pu  L0=0.5  Saturation=[ 0,0 ; 0.0024,1.2 ; 1.0,1.52 ]  InitialFluxes=[-1.0109960716468 0.506091473811006 0.504904597835851]  MoreParameters=off  BreakLoop=off  DataType=off  TransfoNumber=1
  Pinit : Constant  Value=P0
  Source_For_LF : powerlib/Electrical Sources/Three-Phase Source  Commented=on  InternalConnection=Yg  VoltagePhases=off  Voltage=(400000)*1.0018  PhaseAngle=1.1424  Voltage_phases=[25e3 25e3 25e3]/sqrt(3)  PhaseAngles_phases=[0 -120 +120]  Frequency=50  NonIdealSource=off  SpecifyImpedance=off  Resistance=0  Inductance=0  ShortCircuitLevel=100e6  BaseVoltage=Un  XRratio=7  BusType=PQ  Pref=P0*Sb  Qref=Q0*Sb  Prefabc=[10e3, 10e3, 10e3]  Qrefabc=[0, 0, 0]  Qmin=-inf  Qmax=inf
  Vvsc_init : Constant  Value=Vvsc0
  mp3 : Gain  Gain=Vb
  A : PMIOPort  Port=1  Side=Right
  B : PMIOPort  Port=2  Side=Right
  C : PMIOPort  Port=3  Side=Right
  m : Outport
  wires:
  Add/1 -> Control loops/2(P_set)
  dE_set (pu)/1 -> Add1/1
  Bus1/1 -> [eg_meas]
  Add1/1 -> Control loops/1(E_set)
  Vvsc_init/1 -> Add1/2
  Pinit/1 -> Add/2
  dP_set (pu)/1 -> Add/1
  Bus10/1 -> [vg_meas]
  Bus2/1 -> [is_meas]
  Memory2/1 -> Mean_model/1(Uref)
  Bus10/2 -> [ig_meas]
  [is_meas] -> 1/Ib5/1
  1/Ib1/1 -> Control loops/5(ig_abc_pu), Bus Creator/3  "ig_pu"
  [ig_meas] -> 1/Ib1/1
  [vg_meas] -> 1/Ib3/1
  1/Ib3/1 -> Bus Creator/2, Control loops/3(vg_abc_pu)  "vg_pu"
  Control loops/2(m) -> Bus Creator/1  "control"
  Bus Creator/1 -> m/1
  [eg_meas] -> 1/Ib2/1
  1/Ib2/1 -> Control loops/4(eg_abc_pu)
  1/Ib5/1 -> Control loops/6(is_abc_pu), Bus Creator/4  "is_pu"
  Control loops/1(vm_abc_ref_pu) -> mp3/1
  mp3/1 -> Memory2/1
  connections:
  DC Voltage Source/RConn1 -- Mean_model/LConn1
  DC Voltage Source/LConn1 -- Mean_model/LConn2
  Bus1/LConn1 -- Output_Filter/RConn1
  Bus1/LConn2 -- Output_Filter/RConn2
  Bus1/LConn3 -- Output_Filter/RConn3
  Output_Transformer/LConn1 -- Bus1/RConn1
  Bus1/RConn2 -- Output_Transformer/LConn2
  Bus1/RConn3 -- Output_Transformer/LConn3
  Bus10/LConn1 -- Output_Transformer/RConn1
  Bus10/LConn2 -- Output_Transformer/RConn2
  Bus10/LConn3 -- Output_Transformer/RConn3
  C/RConn1 -- Source_For_LF/RConn3 -- Bus10/RConn3
  B/RConn1 -- Source_For_LF/RConn2 -- Bus10/RConn2
  A/RConn1 -- Load Flow Bus/LConn1 -- Source_For_LF/RConn1 -- Bus10/RConn1
  Bus2/LConn1 -- Mean_model/RConn1
  Bus2/LConn2 -- Mean_model/RConn2
  Bus2/LConn3 -- Mean_model/RConn3
  Bus2/RConn1 -- Output_Filter/LConn1
  Bus2/RConn2 -- Output_Filter/LConn2
  Bus2/RConn3 -- Output_Filter/LConn3

== system VSC_GFo_Variable_Frequency_LCL/Inertial Voltage Source/Mean_model ==
  u_abc : Inport
  Controlled Voltage Source1 : powerlib/Electrical Sources/Controlled Voltage Source  Initialize=on  Source_Type=AC  Amplitude=e0*sqrt(2)  Phase=0  Frequency=fb  Measurements=None
  Controlled Voltage Source2 : powerlib/Electrical Sources/Controlled Voltage Source  Initialize=on  Source_Type=AC  Amplitude=e0*sqrt(2)  Phase=-240  Frequency=fb  Measurements=None
  Controlled Voltage Source4 : powerlib/Electrical Sources/Controlled Voltage Source  Initialize=on  Source_Type=AC  Amplitude=e0*sqrt(2)  Phase=-120  Frequency=fb  Measurements=None
  Demux : Demux  Outputs=3
  Ground2 : powerlib/Elements/Ground  LConnTagsString=a
  A : PMIOPort  Port=1  Side=Right
  B : PMIOPort  Port=2  Side=Right
  C : PMIOPort  Port=3  Side=Right
  wires:
  u_abc/1 -> Demux/1
  Demux/2 -> Controlled Voltage Source4/1
  Demux/3 -> Controlled Voltage Source2/1
  Demux/1 -> Controlled Voltage Source1/1
  connections:
  Controlled Voltage Source4/LConn1 -- Controlled Voltage Source1/LConn1 -- Controlled Voltage Source2/LConn1 -- Ground2/LConn1
  Controlled Voltage Source2/RConn1 -- C/RConn1
  Controlled Voltage Source4/RConn1 -- B/RConn1
  Controlled Voltage Source1/RConn1 -- A/RConn1

== system VSC_GFo_Variable_Frequency_LCL/Inertial Voltage Source/Simplified SG ==
  eg_mes : Inport
  ig_mes : Inport  Port=2
  E_set : Inport  Port=3
  " Active & Reactive Power" : Subsystem  DialogController=POWERSYS.PowerSysDialog
  Bus Creator : BusCreator  Inputs=2
  Mux : Mux  Inputs=3
  Power control1 : Subsystem
  Signal Conversion : SignalConversion  OverrideOpt=off
  pu --> SI : Subsystem
  vg_abc : Outport
  m : Outport  Port=2
  wires:
  pu --> SI/1(e_a_SI) -> Mux/1
  ig_mes/1 -> " Active & Reactive Power"/2(Ig_abc)
  eg_mes/1 -> " Active & Reactive Power"/1(e_abc)
  Power control1/3(v_c) -> pu --> SI/3(e_c_pu)
  Mux/1 -> vg_abc/1
  pu --> SI/3(e_c_SI) -> Mux/3
  " Active & Reactive Power"/1(P) -> Power control1/1(P_meas)
  pu --> SI/2(e_b_SI) -> Mux/2
  Power control1/1(v_a) -> pu --> SI/1(e_a_pu)
  Power control1/2(v_b) -> pu --> SI/2(e_b_pu)
  E_set/1 -> Power control1/2(E_set)
  Signal Conversion/1 -> m/1
  Bus Creator/1 -> Signal Conversion/1
  [P_meas] -> Bus Creator/1  "P"
  Power control1/4(f_pu) -> Bus Creator/2  "f"

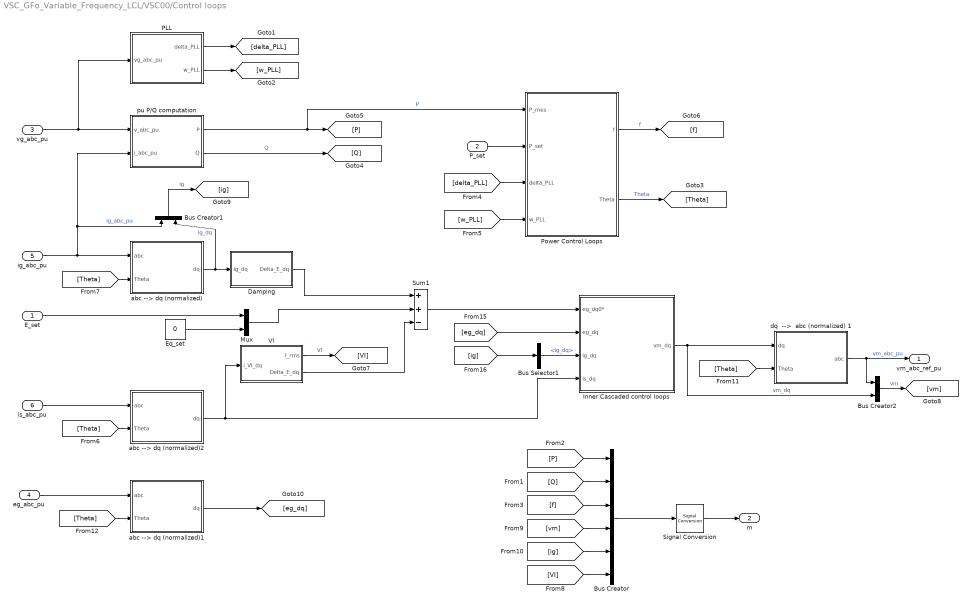
== system VSC_GFo_Variable_Frequency_LCL/VSC00/Control loops ==
  E_set : Inport
  P_set : Inport  Port=2
  vg_abc_pu : Inport  Port=3
  eg_abc_pu : Inport  Port=4
  ig_abc_pu : Inport  Port=5
  is_abc_pu : Inport  Port=6
  " pu P/Q computation" : Subsystem  DialogController=POWERSYS.PowerSysDialog
  Bus Creator : BusCreator  Inputs=6
  Bus Creator1 : BusCreator  Inputs=2
  Bus Creator2 : BusCreator  Inputs=2
  Bus Selector1 : BusSelector  OutputSignals=ig_dq
  Damping : Subsystem
  Eq_set : Constant  Value=0
  Inner Cascaded control loops : Subsystem
  Mux : Mux  Inputs=2
  PLL : Subsystem
  Power Control Loops : Subsystem
  Signal Conversion : SignalConversion  OverrideOpt=off
  Sum1 : Sum  Inputs=++-
  VI : Subsystem
  abc --> dq (normalized) : Subsystem
  abc --> dq (normalized)1 : Subsystem
  abc --> dq (normalized)2 : Subsystem
  dq  -->  abc (normalized) 1 : Subsystem
  vm_abc_ref_pu : Outport
  m : Outport  Port=2
  wires:
  Signal Conversion/1 -> m/1
  [P] -> Bus Creator/1
  [Q] -> Bus Creator/2
  [f] -> Bus Creator/3
  E_set/1 -> Mux/1
  " pu P/Q computation"/2(Q) -> [Q]  "Q"
  [delta_PLL] -> Power Control Loops/3(delta_PLL)
  P_set/1 -> Power Control Loops/2(P_set)
  [w_PLL] -> Power Control Loops/4(w_PLL)
  Power Control Loops/1(f) -> [f]  "f"
  PLL/1(delta_PLL) -> [delta_PLL]
  PLL/2(w_PLL) -> [w_PLL]
  " pu P/Q computation"/1(P) -> Power Control Loops/1(P_mes), [P]  "P"
  ig_abc_pu/1 -> Bus Creator1/1, " pu P/Q computation"/2(i_abc_pu), abc --> dq (normalized)/1(abc)  "ig_abc_pu"
  abc --> dq (normalized)/1(dq) -> Damping/1(ig_dq), Bus Creator1/2  "ig_dq"
  Power Control Loops/2(Theta) -> [Theta]  "Theta"
  [Theta] -> abc --> dq (normalized)/2(Theta)
  VI/2(Delta_E_dq) -> Sum1/3
  Damping/1("Delta_E_dq ") -> Sum1/1
  VI/1(I_rms) -> [VI]  "VI"
  Mux/1 -> Sum1/2
  Eq_set/1 -> Mux/2
  [vm] -> Bus Creator/4
  [VI] -> Bus Creator/6
  Bus Creator/1 -> Signal Conversion/1
  Bus Creator1/1 -> [ig]  "ig"
  [ig] -> Bus Creator/5
  [Theta] -> abc --> dq (normalized)2/2(Theta)
  vg_abc_pu/1 -> PLL/1(vg_abc_pu), " pu P/Q computation"/1(v_abc_pu)
  abc --> dq (normalized)2/1(dq) -> Inner Cascaded control loops/4(is_dq), VI/1(i_VI_dq)
  [Theta] -> abc --> dq (normalized)1/2(Theta)
  abc --> dq (normalized)1/1(dq) -> [eg_dq]
  is_abc_pu/1 -> abc --> dq (normalized)2/1(abc)
  eg_abc_pu/1 -> abc --> dq (normalized)1/1(abc)
  [eg_dq] -> Inner Cascaded control loops/2(eg_dq)
  Inner Cascaded control loops/1(vm_dq) -> dq  -->  abc (normalized) 1/1(dq), Bus Creator2/2  "vm_dq"
  dq  -->  abc (normalized) 1/1(abc) -> Bus Creator2/1, vm_abc_ref_pu/1  "vm_abc_pu"
  [Theta] -> dq  -->  abc (normalized) 1/2(Theta)
  Bus Creator2/1 -> [vm]  "vm"
  Bus Selector1/1 -> Inner Cascaded control loops/3(ig_dq)  "<ig_dq>"
  [ig] -> Bus Selector1/1
  Sum1/1 -> Inner Cascaded control loops/1(eg_dq0*)

== system VSC_GFo_Variable_Frequency_LCL/VSC00/Mean_model ==
  Uref : Inport
  NOT1 : Logic  Operator=NOT  IconShape=distinctive  AllPortsSameDT=off  OutDataTypeStr=boolean
  Scope : Scope
  Step1 : Step  Time=Time_Step  SampleTime=Time_Step
  Three-Phase Breaker1 : powerlib/Elements/Three-Phase Breaker  InitialState=closed  SwitchA=on  SwitchB=on  SwitchC=on  SwitchTimes="[4/60  10/60]"  External=on  BreakerResistance=0.001  SnubberResistance=1e6  SnubberCapacitance=inf  Measurements=None
  Three-Phase Breaker2 : powerlib/Elements/Three-Phase Breaker  InitialState=open  SwitchA=on  SwitchB=on  SwitchC=on  SwitchTimes="[4/60  10/60]"  External=on  BreakerResistance=0.001  SnubberResistance=1e6  SnubberCapacitance=inf  Measurements=None
  Three-Phase Source : powerlib/Electrical Sources/Three-Phase Source  InternalConnection=Yg  VoltagePhases=off  Voltage=Vvsc0*Un1  PhaseAngle=Theta_vsc0  Voltage_phases=[25e3 25e3 25e3]/sqrt(3)  PhaseAngles_phases=[0 -120 +120]  Frequency=50  NonIdealSource=off  SpecifyImpedance=off  Resistance=0  Inductance=0  ShortCircuitLevel=100e6  BaseVoltage=VSC01_Un1  XRratio=7  BusType=swing  Pref=0.3  Qref=0  Prefabc=[10e3, 10e3, 10e3]  Qrefabc=[0, 0, 0]  Qmin=-Inf  Qmax=Inf
  Universal Bridge : powerlib/Power Electronics/Universal Bridge  Arms=3  SnubberResistance=1e5  SnubberCapacitance=inf  Device=Average-model based VSC  Ron=1e-3  Lon=0  ForwardVoltages="[  0  0  ]"  ForwardVoltage=0  GTOparameters=[ 10e-6 , 20e-6 ]  IGBTparameters=[ 1e-6 , 2e-6 ]  Measurements=None  Measurements_2=None  converterType=Rectifier
  Vdc : powerlib/Measurements/Voltage Measurement  PhasorSimulation=off  OutputType=Complex  PSBequivalent=0
  mp3 : Gain  Gain=2/VSC01_Udcb
  PhA : PMIOPort  Port=1  Side=Right
  PhB : PMIOPort  Port=2  Side=Right
  PhC : PMIOPort  Port=3  Side=Right
  Vdc+ : PMIOPort  Port=4  Side=Left
  Vdc- : PMIOPort  Port=5  Side=Left
  wires:
  Vdc/1 -> Scope/1
  Uref/1 -> mp3/1
  mp3/1 -> Universal Bridge/1
  Step1/1 -> Three-Phase Breaker2/1, NOT1/1
  NOT1/1 -> Three-Phase Breaker1/1
  connections:
  Vdc-/RConn1 -- Universal Bridge/RConn2 -- Vdc/LConn2
  Vdc+/RConn1 -- Universal Bridge/RConn1 -- Vdc/LConn1
  Three-Phase Source/RConn3 -- Three-Phase Breaker1/RConn3
  Three-Phase Source/RConn2 -- Three-Phase Breaker1/RConn2
  Three-Phase Source/RConn1 -- Three-Phase Breaker1/RConn1
  Three-Phase Breaker2/RConn3 -- Universal Bridge/LConn3
  Three-Phase Breaker2/RConn2 -- Universal Bridge/LConn2
  Three-Phase Breaker2/RConn1 -- Universal Bridge/LConn1
  PhC/RConn1 -- Three-Phase Breaker1/LConn3 -- Three-Phase Breaker2/LConn3
  PhB/RConn1 -- Three-Phase Breaker1/LConn2 -- Three-Phase Breaker2/LConn2
  PhA/RConn1 -- Three-Phase Breaker1/LConn1 -- Three-Phase Breaker2/LConn1

== system VSC_GFo_Variable_Frequency_LCL/VSC00/Output_Filter ==
  Filter capacitance : powerlib/Elements/Three-Phase Series RLC Branch  LConnTagsString=A|B|C  RConnTagsString=A|B|C  BranchType=C  Resistance=0  Inductance=C_line(1)  Capacitance=Cf_pu*Cb  Measurements=None
  Filter inductance : powerlib/Elements/Three-Phase Series RLC Branch  LConnTagsString=A|B|C  RConnTagsString=A|B|C  BranchType=RL  Resistance=Rf_pu*Zb  Inductance=Lf_pu*Lb  Capacitance=1e-6  Measurements=None
  Ground : powerlib/Elements/Ground  LConnTagsString=a
  A : PMIOPort  Port=1  Side=Left
  a : PMIOPort  Port=2  Side=Right
  B : PMIOPort  Port=3  Side=Left
  b : PMIOPort  Port=4  Side=Right
  C : PMIOPort  Port=5  Side=Left
  c : PMIOPort  Port=6  Side=Right
  connections:
  Filter inductance/RConn1 -- Filter capacitance/LConn1 -- a/RConn1
  Filter inductance/RConn3 -- Filter capacitance/LConn3 -- c/RConn1
  Filter inductance/LConn2 -- B/RConn1
  Filter inductance/LConn3 -- C/RConn1
  Filter inductance/LConn1 -- A/RConn1
  Filter inductance/RConn2 -- Filter capacitance/LConn2 -- b/RConn1
  Filter capacitance/RConn2 -- Filter capacitance/RConn3 -- Filter capacitance/RConn1 -- Ground/LConn1

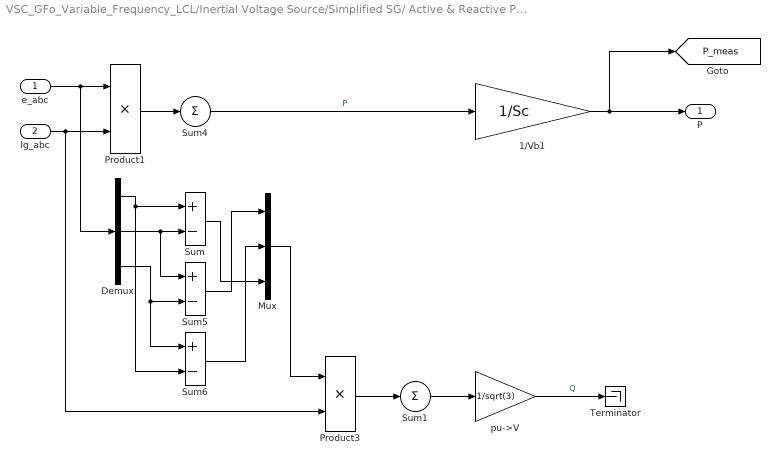
== system VSC_GFo_Variable_Frequency_LCL/Inertial Voltage Source/Simplified SG/ Active & Reactive Power ==
  e_abc : Inport  PortDimensions=3
  Ig_abc : Inport  Port=2  PortDimensions=3
  1/Vb1 : Gain  Gain=1/Sc
  Demux : Demux  Outputs=3
  Mux : Mux  Inputs=3
  Product1 : Product  SaturateOnIntegerOverflow=on  InputSameDT=on  OutDataTypeStr=Inherit: Same as first input
  Product3 : Product  SaturateOnIntegerOverflow=on  InputSameDT=on  OutDataTypeStr=Inherit: Same as first input
  Sum : Sum  Inputs=+-  SaturateOnIntegerOverflow=on  InputSameDT=on  OutDataTypeStr=Inherit: Same as first input
  Sum1 : Sum  Inputs=1  SaturateOnIntegerOverflow=on  InputSameDT=on  OutDataTypeStr=Inherit: Same as first input
  Sum4 : Sum  Inputs=1  SaturateOnIntegerOverflow=on  InputSameDT=on  OutDataTypeStr=Inherit: Same as first input
  Sum5 : Sum  Inputs=+-  SaturateOnIntegerOverflow=on  InputSameDT=on  OutDataTypeStr=Inherit: Same as first input
  Sum6 : Sum  Inputs=+-  SaturateOnIntegerOverflow=on  InputSameDT=on  OutDataTypeStr=Inherit: Same as first input
  Terminator : Terminator
  pu->V : Gain  Gain=1/sqrt(3)  SaturateOnIntegerOverflow=on  OutDataTypeStr=Inherit: Same as input  ParamDataTypeStr=Inherit: Same as input
  P : Outport
  tag scope: P_meas=global
  wires:
  Mux/1 -> Product3/1
  Sum6/1 -> Mux/2
  Sum5/1 -> Mux/1
  Sum/1 -> Mux/3
  Demux/3 -> Sum6/1, Sum5/2
  Demux/2 -> Sum5/1, Sum/2
  Demux/1 -> Sum6/2, Sum/1
  Sum4/1 -> 1/Vb1/1  "P"
  Ig_abc/1 -> Product3/2, Product1/2
  e_abc/1 -> Demux/1, Product1/1
  Product1/1 -> Sum4/1
  Product3/1 -> Sum1/1
  Sum1/1 -> pu->V/1
  pu->V/1 -> Terminator/1  "Q"
  1/Vb1/1 -> [P_meas], P/1

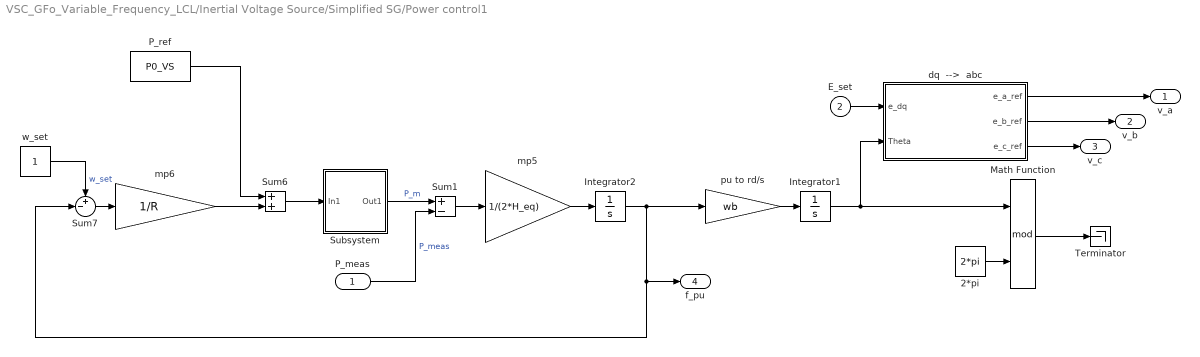
== system VSC_GFo_Variable_Frequency_LCL/Inertial Voltage Source/Simplified SG/Power control1 ==
  P_meas : Inport
  E_set : Inport  Port=2
  " pu to rd/s" : Gain  Gain=wb
  2*pi : Constant  Value=2*pi
  Integrator1 : Integrator
  Integrator2 : Integrator  InitialCondition=1
  Math Function : Math  Operator=mod  SaturateOnIntegerOverflow=on
  P_ref : Constant  Value=P0_VS
  Subsystem : Subsystem
  Sum1 : Sum  Inputs=+-
  Sum6 : Sum
  Sum7 : Sum  Inputs=+-|
  Terminator : Terminator
  "dq  -->  abc " : Subsystem
  mp5 : Gain  Gain=1/(2*H_eq)
  mp6 : Gain  Gain=1/R
  w_set : Constant
  v_a : Outport
  v_b : Outport  Port=2
  v_c : Outport  Port=3
  f_pu : Outport  Port=4
  wires:
  Integrator1/1 -> "dq  -->  abc "/2(Theta), Math Function/1
  " pu to rd/s"/1 -> Integrator1/1
  Math Function/1 -> Terminator/1
  2*pi/1 -> Math Function/2
  "dq  -->  abc "/1(e_a_ref) -> v_a/1
  "dq  -->  abc "/2(e_b_ref) -> v_b/1
  "dq  -->  abc "/3(e_c_ref) -> v_c/1
  w_set/1 -> Sum7/1  "w_set"
  E_set/1 -> "dq  -->  abc "/1(e_dq)
  Sum7/1 -> mp6/1
  P_ref/1 -> Sum6/1
  Integrator2/1 -> " pu to rd/s"/1, f_pu/1, Sum7/2
  Sum1/1 -> mp5/1
  P_meas/1 -> Sum1/2  "P_meas"
  mp6/1 -> Sum6/2
  Sum6/1 -> Subsystem/1(In1)
  Subsystem/1(Out1) -> Sum1/1  "P_m"
  mp5/1 -> Integrator2/1

== system VSC_GFo_Variable_Frequency_LCL/Inertial Voltage Source/Simplified SG/pu --> SI ==
  e_a_pu : Inport
  e_b_pu : Inport  Port=2
  e_c_pu : Inport  Port=3
  nq : Gain  Gain=Vb
  nq1 : Gain  Gain=Vb
  nq2 : Gain  Gain=Vb
  e_a_SI : Outport
  e_b_SI : Outport  Port=2
  e_c_SI : Outport  Port=3
  wires:
  e_b_pu/1 -> nq1/1
  nq2/1 -> e_c_SI/1
  nq/1 -> e_a_SI/1
  e_c_pu/1 -> nq2/1
  nq1/1 -> e_b_SI/1
  e_a_pu/1 -> nq/1

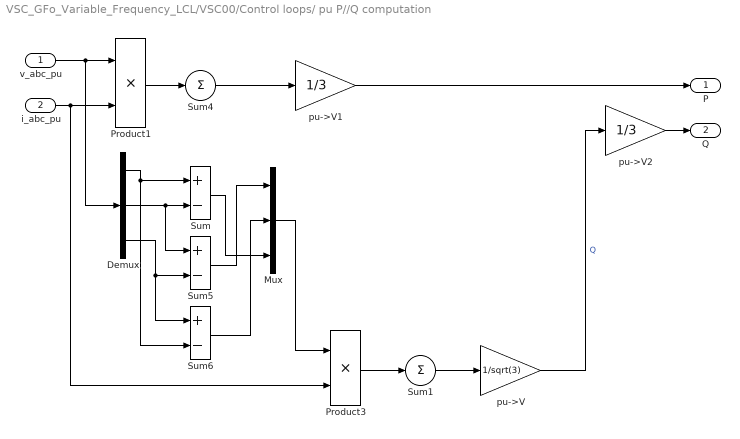
== system VSC_GFo_Variable_Frequency_LCL/VSC00/Control loops/ pu P//Q computation ==
  v_abc_pu : Inport  PortDimensions=3
  i_abc_pu : Inport  Port=2  PortDimensions=3
  Demux : Demux  Outputs=3
  Mux : Mux  Inputs=3
  Product1 : Product  SaturateOnIntegerOverflow=on  InputSameDT=on  OutDataTypeStr=Inherit: Same as first input
  Product3 : Product  SaturateOnIntegerOverflow=on  InputSameDT=on  OutDataTypeStr=Inherit: Same as first input
  Sum : Sum  Inputs=+-  SaturateOnIntegerOverflow=on  InputSameDT=on  OutDataTypeStr=Inherit: Same as first input
  Sum1 : Sum  Inputs=1  SaturateOnIntegerOverflow=on  InputSameDT=on  OutDataTypeStr=Inherit: Same as first input
  Sum4 : Sum  Inputs=1  SaturateOnIntegerOverflow=on  InputSameDT=on  OutDataTypeStr=Inherit: Same as first input
  Sum5 : Sum  Inputs=+-  SaturateOnIntegerOverflow=on  InputSameDT=on  OutDataTypeStr=Inherit: Same as first input
  Sum6 : Sum  Inputs=+-  SaturateOnIntegerOverflow=on  InputSameDT=on  OutDataTypeStr=Inherit: Same as first input
  pu->V : Gain  Gain=1/sqrt(3)  SaturateOnIntegerOverflow=on  OutDataTypeStr=Inherit: Same as input  ParamDataTypeStr=Inherit: Same as input
  pu->V1 : Gain  Gain=1/3  SaturateOnIntegerOverflow=on  OutDataTypeStr=Inherit: Same as input  ParamDataTypeStr=Inherit: Same as input
  pu->V2 : Gain  Gain=1/3  SaturateOnIntegerOverflow=on  OutDataTypeStr=Inherit: Same as input  ParamDataTypeStr=Inherit: Same as input
  P : Outport
  Q : Outport  Port=2
  wires:
  pu->V/1 -> pu->V2/1  "Q"
  Mux/1 -> Product3/1
  Sum6/1 -> Mux/2
  Sum5/1 -> Mux/1
  Sum/1 -> Mux/3
  Demux/3 -> Sum6/1, Sum5/2
  Demux/2 -> Sum5/1, Sum/2
  Demux/1 -> Sum6/2, Sum/1
  Sum4/1 -> pu->V1/1
  i_abc_pu/1 -> Product3/2, Product1/2
  v_abc_pu/1 -> Demux/1, Product1/1
  Product1/1 -> Sum4/1
  Product3/1 -> Sum1/1
  Sum1/1 -> pu->V/1
  pu->V1/1 -> P/1
  pu->V2/1 -> Q/1

== system VSC_GFo_Variable_Frequency_LCL/VSC00/Control loops/Damping ==
  ig_dq : Inport
  Filter w_LF : Subsystem
      mask Display: disp('\omega_{LF} / (s + \omega_{LF})','texmode','on')
  Sum5 : Sum  Inputs=|+-
  nq1 : Gain  Gain=Rv
  "Delta_E_dq " : Outport
  wires:
  ig_dq/1 -> nq1/1
  Sum5/1 -> "Delta_E_dq "/1
  Filter w_LF/1(s) -> Sum5/1
  nq1/1 -> Sum5/2, Filter w_LF/1(e)

== system VSC_GFo_Variable_Frequency_LCL/VSC00/Control loops/Inner Cascaded control loops ==
  eg_dq0* : Inport
  eg_dq : Inport  Port=2
  ig_dq : Inport  Port=3
  is_dq : Inport  Port=4
  Amplitude : Subsystem
  Compare To Constant : simulink/Logic and Bit Operations/Compare To Constant  relop=<=  const=I_max  OutDataTypeStr=boolean
  Current PI control : Subsystem
      mask Display:
      | plot(0,0,100,100, [10,10,90,90,10,40,40,10,90,60,60,90],[90,10,10,90,90,60,40,10,10,40,60,90])
      | disp('PI')
  Memory : Memory
  Voltage PI control : Subsystem
      mask Display:
      | plot(0,0,100,100, [10,10,90,90,10,40,40,10,90,60,60,90],[90,10,10,90,90,60,40,10,10,40,60,90])
      | disp('PI')
  w_pu : Constant
  vm_dq : Outport
  wires:
  Amplitude/2(cond) -> Compare To Constant/1
  eg_dq0*/1 -> Voltage PI control/2(Eg_dq0*)
  Voltage PI control/1(Is_dq0*) -> Amplitude/1(is_unsat)
  Amplitude/1(is_sat) -> Current PI control/3(Is_dq0*)
  w_pu/1 -> Current PI control/4(w), Voltage PI control/4(w)
  Current PI control/1(Vm_dq0*) -> vm_dq/1
  is_dq/1 -> Current PI control/1(Is_dq0)
  eg_dq/1 -> Current PI control/2(Eg_dq0), Voltage PI control/1(Eg_dq0)
  ig_dq/1 -> Voltage PI control/3(Ig_dq0)
  Compare To Constant/1 -> Memory/1
  Memory/1 -> Voltage PI control/5(block integ)

== system VSC_GFo_Variable_Frequency_LCL/VSC00/Control loops/PLL ==
  vg_abc_pu : Inport
  Demux : Demux  Outputs=2
  PI PLL controller : Subsystem
  Terminator : Terminator
  abc --> dq (normalized) : Subsystem
  delta_PLL : Outport
  w_PLL : Outport  Port=2
  wires:
  Demux/2 -> PI PLL controller/1(Vq)
  PI PLL controller/1(w_PLL) -> w_PLL/1
  Demux/1 -> Terminator/1
  PI PLL controller/2(delta_theta) -> abc --> dq (normalized)/2(Theta), delta_PLL/1
  vg_abc_pu/1 -> abc --> dq (normalized)/1(abc)
  abc --> dq (normalized)/1(dq) -> Demux/1

== system VSC_GFo_Variable_Frequency_LCL/VSC00/Control loops/Power Control Loops ==
  P_mes : Inport
  P_set : Inport  Port=2
  delta_PLL : Inport  Port=3
  w_PLL : Inport  Port=4
  Merge : Merge  Inputs=3
  Merge1 : Merge  Inputs=3
  Power control loops : Subsystem
  Strategy 1 : Subsystem
  Strategy 2 : Subsystem
  Switch Case : SwitchCase  CaseConditions={1,2,3}  ShowDefaultCase=off
  w_set2 : Constant  Value=gainpopup
  w_set_pu : Constant
  f : Outport
  Theta : Outport  Port=2
  wires:
  w_set2/1 -> Switch Case/1
  P_mes/1 -> Power control loops/1(P_mes), Strategy 2/1(P_mes), Strategy 1/1(P_mes)
  P_set/1 -> Strategy 2/2(P_set), Power control loops/2(P_set), Strategy 1/2(P_set)
  delta_PLL/1 -> Strategy 1/3(delta_PLL)
  w_PLL/1 -> Strategy 2/3(w_PLL), Strategy 1/4(w_PLL)
  Switch Case/1 -> Strategy 1/Action
  Switch Case/2 -> Strategy 2/Action
  w_set_pu/1 -> Power control loops/3(w_set_pu)
  Switch Case/3 -> Power control loops/Action
  Strategy 1/1(frequency) -> Merge/1
  Strategy 2/1(frequency) -> Merge/2
  Power control loops/1(frequency) -> Merge/3
  Strategy 1/2(theta) -> Merge1/1
  Strategy 2/2(theta) -> Merge1/2
  Power control loops/2(theta) -> Merge1/3
  Merge/1 -> f/1
  Merge1/1 -> Theta/1

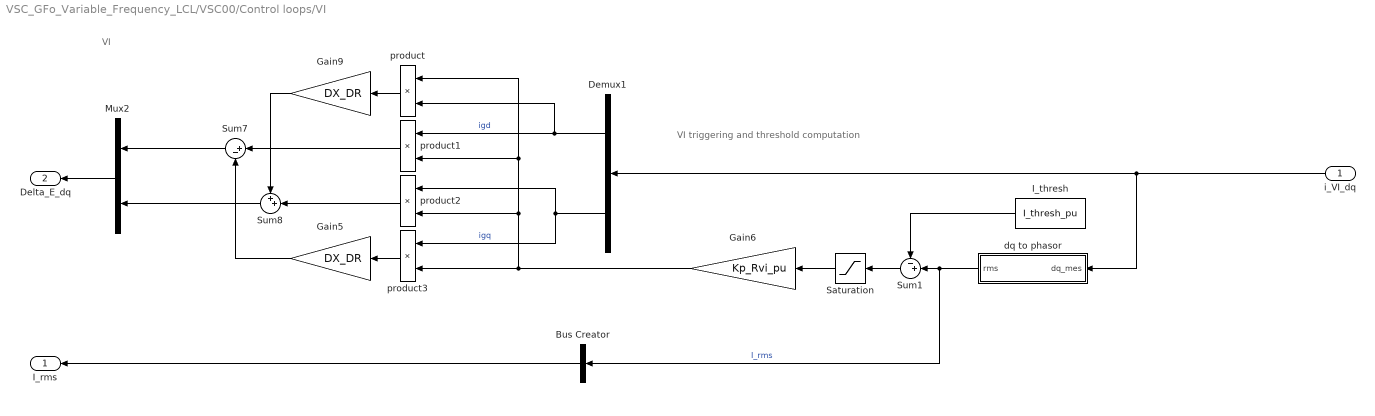
== system VSC_GFo_Variable_Frequency_LCL/VSC00/Control loops/VI ==
  note: VI
  note: VI triggering and threshold computation
  i_VI_dq : Inport
  Bus Creator : BusCreator  Inputs=1
  Demux1 : Demux  Outputs=2
  Gain5 : Gain  Gain=DX_DR
  Gain6 : Gain  Gain=Kp_Rvi_pu
  Gain9 : Gain  Gain=DX_DR
  I_thresh : Constant  Value=I_thresh_pu
  Mux2 : Mux  Inputs=2
  Saturation : Saturate  UpperLimit=inf  LowerLimit=0
  Sum1 : Sum  Inputs=-+|
  Sum7 : Sum  Inputs=|+-
  Sum8 : Sum  Inputs=++|
  dq to phasor : Subsystem
  product{,1..3} (4 alike) : Product  SaturateOnIntegerOverflow=on  RndMeth=Zero  InputSameDT=on  OutDataTypeStr=Inherit: Same as first input
  I_rms : Outport
  Delta_E_dq : Outport  Port=2
  wires:
  i_VI_dq/1 -> Demux1/1, dq to phasor/1(dq_mes)
  Sum8/1 -> Mux2/2
  Sum7/1 -> Mux2/1
  product2/1 -> Sum8/2
  Gain9/1 -> Sum8/1
  Gain5/1 -> Sum7/2
  product1/1 -> Sum7/1
  Demux1/2 -> product3/1, product2/1  "igq"
  Demux1/1 -> product/2, product1/1  "igd"
  product/1 -> Gain9/1
  product3/1 -> Gain5/1
  Gain6/1 -> product2/2, product1/2, product/1, product3/2
  Mux2/1 -> Delta_E_dq/1
  I_thresh/1 -> Sum1/1
  Saturation/1 -> Gain6/1
  dq to phasor/1(rms) -> Bus Creator/1, Sum1/2  "I_rms"
  Sum1/1 -> Saturation/1
  Bus Creator/1 -> I_rms/1
